simulink model "dcmotortest"  (R2016a)
settings: Solver=VariableStepAuto  StartTime=0.0  StopTime=1  RelTol=1e-3
values from neighbouring files (symbols this model uses):
  MR_Kp = 2*MR_L/MR_Tau - MR_R    (= 4.46666666667)    [ControllerDesign.m]
  MR_L = 8.62835e-4    (= 0.000862835)    [ControllerDesign.m]
  MR_R = 6.7    [ControllerDesign.m]
  Vmax = 12    [ControllerDesign.m]
libraries: simulink x1, cstblocks x1
settings Model: Creator=masom  LastModifiedBy=masom

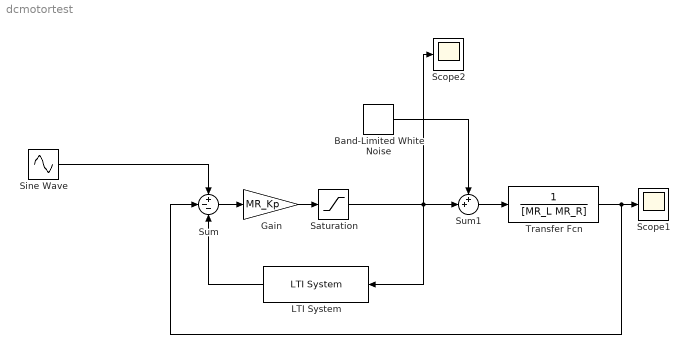
== system dcmotortest ==
  Band-Limited White Noise : simulink/Sources/Band-Limited White Noise  Cov=0.001  Ts=0.1  seed=[23341]
  Gain : Gain  Gain=MR_Kp
  LTI System : cstblocks/LTI System  sys=MR_ctrl  IC=[]
  Saturation : Saturate  UpperLimit=Vmax  LowerLimit=-Vmax
  Scope1 : Scope
  Scope2 : Scope
  Sine Wave : Sin  Amplitude=4  Frequency=100  SampleTime=0
  Sum : Sum  Inputs=+--
  Sum1 : Sum  Inputs=++|
  Transfer Fcn : TransferFcn  Denominator=[MR_L MR_R]
  wires:
  Gain/1 -> Saturation/1
  Transfer Fcn/1 -> Scope1/1, Sum/2
  Sum/1 -> Gain/1
  LTI System/1 -> Sum/3
  Saturation/1 -> Sum1/2, Scope2/1, LTI System/1
  Sine Wave/1 -> Sum/1
  Sum1/1 -> Transfer Fcn/1
  Band-Limited White Noise/1 -> Sum1/1
